simulink model "DC_Motor"  (R2017b)
settings: Solver=VariableStepAuto  StartTime=0.0  StopTime=10.0  RelTol=1e-3
values from neighbouring files (symbols this model uses):
  B1 = [0; B]    [Ch8_24.m]    (also in Ch8_26.m = [0 ; 1]; DC_Model.m = [0; 0; 1/L])
  J = 31*10^(-6)    (= 3.1e-05)    [DC_Model.m]
  Ke = 0.54    [DC_Model.m]
  Kt = 0.54    [DC_Model.m]
  L = 0.008    [DC_Model.m]
  R = 2    [Ch8_18.m]    (also in Ch8_26.m = 1; DC_Model.m)
settings Model: Creator=Student_4  LastModifiedBy=Student_4

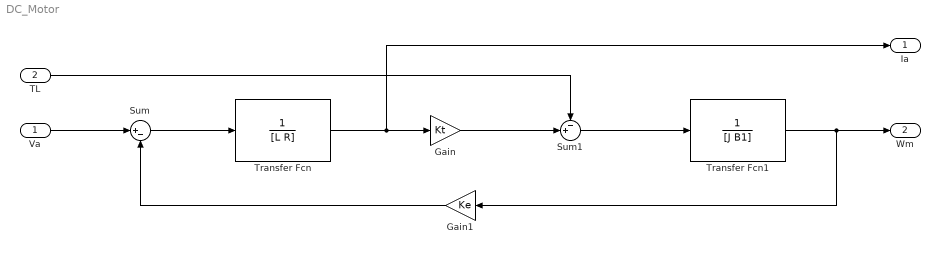
== system DC_Motor ==
  Va : Inport
  TL : Inport  Port=2
  Gain : Gain  Gain=Kt
  Gain1 : Gain  Gain=Ke
  Sum : Sum  Inputs=|+-
  Sum1 : Sum  Inputs=-+|
  Transfer Fcn : TransferFcn  Denominator=[L R]
  Transfer Fcn1 : TransferFcn  Denominator=[J B1]
  Ia : Outport
  Wm : Outport  Port=2
  wires:
  Va/1 -> Sum/1
  Sum/1 -> Transfer Fcn/1
  Transfer Fcn/1 -> Ia/1, Gain/1
  Gain/1 -> Sum1/2
  TL/1 -> Sum1/1
  Sum1/1 -> Transfer Fcn1/1
  Transfer Fcn1/1 -> Gain1/1, Wm/1
  Gain1/1 -> Sum/2
